simulink model "flex2"  (R2021b)
settings: Solver=ode1  StartTime=0.0  StopTime=4  FixedStep=0.001  RelTol=1e-3  EnableMultiTasking=on
values from neighbouring files (symbols this model uses):
  b1 = 0.0085    [part4_prelab.m]    (also in simulation_vs_exp.m; simulation_vs_exp_3_1.m; simulation_vs_exp_3_2.m; simulation_vs_exp_3_3.m)
  b2 = 8.4745E-4    (= 0.00084745)    [part4_prelab.m]    (also in simulation_vs_exp.m; simulation_vs_exp_3_1.m; simulation_vs_exp_3_2.m; simulation_vs_exp_3_3.m)
  c = 4.2    [part4_prelab.m]    (also in simulation_vs_exp.m = 0; simulation_vs_exp_3_1.m = 0; simulation_vs_exp_3_2.m = 0; simulation_vs_exp_3_3.m = 0)
  d1 = 0.5934    [simulation_vs_exp_3_1.m]    (also in simulation_vs_exp_3_2.m; simulation_vs_exp_3_3.m)
  d2 = 0.05934    [simulation_vs_exp_3_1.m]    (also in simulation_vs_exp_3_2.m; simulation_vs_exp_3_3.m)
  k = 0.0351    [part4_prelab.m]    (also in simulation_vs_exp.m; simulation_vs_exp_3_1.m; simulation_vs_exp_3_2.m; simulation_vs_exp_3_3.m)
  kp_notch = 1/amp    [simulation_vs_exp.m]    (also in simulation_vs_exp_3_1.m; simulation_vs_exp_3_2.m; simulation_vs_exp_3_3.m)
  m1 = 2.6634E-4    (= 0.00026634)    [part4_prelab.m]    (also in simulation_vs_exp.m; simulation_vs_exp_3_1.m; simulation_vs_exp_3_2.m; simulation_vs_exp_3_3.m)
  m2 = 1.4383E-4    (= 0.00014383)    [part4_prelab.m]    (also in simulation_vs_exp.m; simulation_vs_exp_3_1.m; simulation_vs_exp_3_2.m; simulation_vs_exp_3_3.m)
  wn = 17.33    [part4_prelab.m]    (also in simulation_vs_exp.m; simulation_vs_exp_3_1.m; simulation_vs_exp_3_2.m; simulation_vs_exp_3_3.m)
  zeta = 0.2669    [part4_prelab.m]    (also in simulation_vs_exp.m; simulation_vs_exp_3_1.m; simulation_vs_exp_3_2.m; simulation_vs_exp_3_3.m)
  zeta_den = 1    [part4_prelab.m]    (also in simulation_vs_exp.m; simulation_vs_exp_3_1.m; simulation_vs_exp_3_2.m; simulation_vs_exp_3_3.m)
undefined symbols (not defined in the file or in its folder): sgn, Ts
libraries: simulink x1
settings Model: SimulationMode=external  ExtModeTrigDuration=50000  Creator=mte360  LastModifiedBy=parth
settings SolverCC: AlgebraicLoopSolver=TrustRegion  PositivePriorityOrder=on
settings DataIOCC: LimitDataPoints=on  MaxDataPoints=100000  SaveFormat=Array  SignalLoggingSaveFormat=ModelDataLogs  ReturnWorkspaceOutputs=off
settings OptimizationCC: ExpressionDepthLimit=2147483647
settings DebuggingCC: UnderspecifiedInitializationDetection=Classic  MergeDetectMultiDrivingBlocksExec=none  SolverPrmCheckMsg=warning  FcnCallInpInsideContextMsg=warning  AllowSymbolicDim=off  StateNameClashWarn=warning  SFUnexpectedBacktrackingDiag=warning  SFNoUnconditionalDefaultTransitionDiag=warning  SFExecutionAtInitializationDiag=none  SFMachineParentedDataDiag=warning  ArithmeticOperatorsInVariantConditions=warning
settings ModelReferenceCC: PropagateSignalLabelsOutOfModel=off
settings SFSimCC: SimUseLocalCustomCode=off  CustomCodeUndefinedFunction=UseInterfaceOnly
settings RTWCC: Description=QUARC Win64 Target Using Toolchain  SystemTargetFile=quarc_win64.tlc  TemplateMakefile=quarc_default_tmf  RTWUseLocalCustomCode=off  Toolchain=QUARC win64 | nmake (64-bit Windows)  BuildConfiguration=Faster Runs
settings CodeAppCC: StateflowObjectComments=on
settings STFCustomTargetCC: ConcurrentExecutionCompliant=on  UseToolchainInfoCompliant=on  SystemTargetFile=quarc_win64.tlc
settings GRTTargetCC: TargetLangStandard=C89/C90 (ANSI)  ParMdlRefBuildCompliant=off  CompOptLevelCompliant=off  CombineOutputUpdateFcns=off  MatFileLogging=off  CPPClassGenCompliant=off  GRTInterface=on  ExtMode=on  ExtModeMexFile=quarc_comm
settings ConfigComp: CovMetricSettings=dw  CovSaveCumulativeToWorkspaceVar=on  CovSaveSingleToWorkspaceVar=on  CovExternalEMLEnable=off

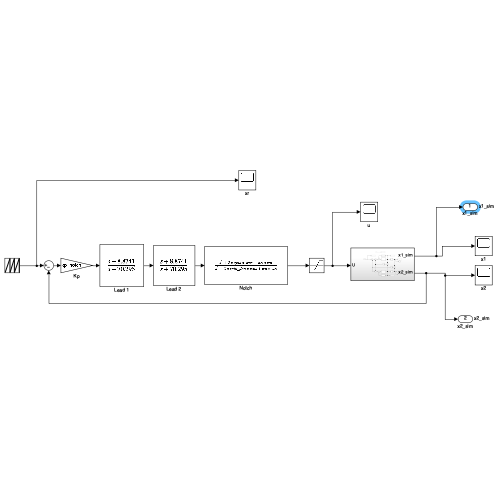
[thumbnail: Simulink's stored preview of the top-level diagram]
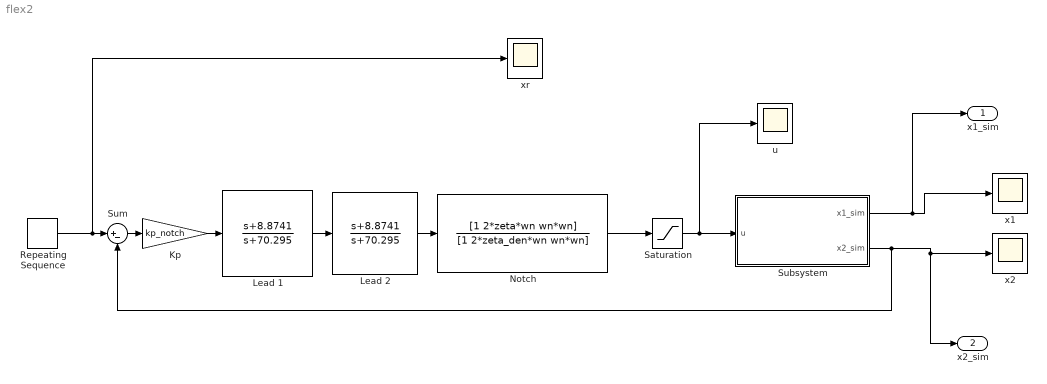
== system flex2 ==
  Kp : Gain  Gain=kp_notch
  Lead 1 : TransferFcn  Numerator=[1 8.8741]  Denominator=[1 70.295]
  Lead 2 : TransferFcn  Numerator=[1 8.8741]  Denominator=[1 70.295]
  Notch : TransferFcn  Numerator=[1 2*zeta*wn wn*wn]  Denominator=[1 2*zeta_den*wn wn*wn]
  Repeating Sequence : simulink/Sources/Repeating Sequence  rep_seq_t=t  rep_seq_y=s
  Saturation : Saturate  UpperLimit=8  LowerLimit=-8
  Subsystem : Subsystem
  Sum : Sum  Inputs=|+-
  u : Scope
  x1 : Scope
  x2 : Scope
  xr : Scope
  x1_sim : Outport  SignalName=x1_sim
  x2_sim : Outport  Port=2  SignalName=x2_sim
  wires:
  Repeating Sequence/1 -> xr/1, Sum/1
  Sum/1 -> Kp/1
  Kp/1 -> Lead 1/1
  Lead 1/1 -> Lead 2/1
  Lead 2/1 -> Notch/1
  Notch/1 -> Saturation/1
  Saturation/1 -> Subsystem/1(u), u/1
  Subsystem/1(x1_sim) -> x1/1, x1_sim/1
  Subsystem/2(x2_sim) -> x2_sim/1, x2/1, Sum/2

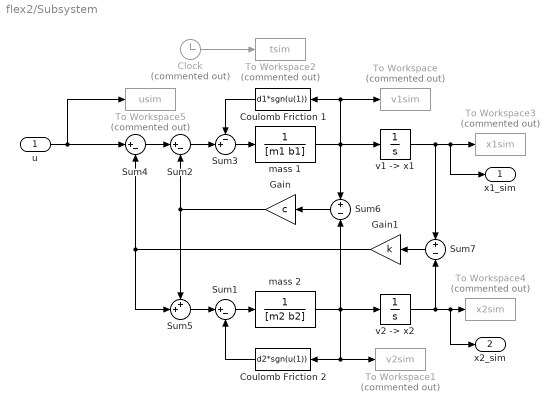
== system flex2/Subsystem ==
  u : Inport
  Clock : Clock  Commented=on
  Coulomb Friction 1 : Fcn  Expr=d1*sgn(u(1))
  Coulomb Friction 2 : Fcn  Expr=d2*sgn(u(1))
  Gain : Gain  Gain=c  SaturateOnIntegerOverflow=on  OutDataTypeStr=Inherit: Same as input  ParamDataTypeStr=Inherit: Same as input
  Gain1 : Gain  Gain=k  SaturateOnIntegerOverflow=on  OutDataTypeStr=Inherit: Same as input  ParamDataTypeStr=Inherit: Same as input
  Sum1 : Sum  Inputs=|+-  SaturateOnIntegerOverflow=on
  Sum2 : Sum  Inputs=|+-  SaturateOnIntegerOverflow=on
  Sum3 : Sum  Inputs=-+|  SaturateOnIntegerOverflow=on
  Sum4 : Sum  Inputs=|+-  SaturateOnIntegerOverflow=on
  Sum5 : Sum  Inputs=++|  SaturateOnIntegerOverflow=on
  Sum6 : Sum  Inputs=+|-  SaturateOnIntegerOverflow=on
  Sum7 : Sum  Inputs=+|-  SaturateOnIntegerOverflow=on
  To Workspace : ToWorkspace  Commented=on  VariableName=v1sim  SampleTime=Ts
  To Workspace1 : ToWorkspace  Commented=on  VariableName=v2sim  SampleTime=Ts
  To Workspace2 : ToWorkspace  Commented=on  VariableName=tsim  SampleTime=Ts
  To Workspace3 : ToWorkspace  Commented=on  VariableName=x1sim  SampleTime=Ts
  To Workspace4 : ToWorkspace  Commented=on  VariableName=x2sim  SampleTime=Ts
  To Workspace5 : ToWorkspace  Commented=on  VariableName=usim  SampleTime=Ts
  mass 1 : TransferFcn  Denominator=[m1 b1]
  mass 2 : TransferFcn  Denominator=[m2 b2]
  "v1 -> x1" : Integrator
  "v2 -> x2" : Integrator
  x1_sim : Outport
  x2_sim : Outport  Port=2
  wires:
  Sum5/1 -> Sum1/1
  Coulomb Friction 1/1 -> Sum3/1
  mass 1/1 -> "v1 -> x1"/1, Sum6/1, Coulomb Friction 1/1, To Workspace/1
  Gain/1 -> Sum2/2, Sum5/1
  Sum2/1 -> Sum3/2
  Sum3/1 -> mass 1/1
  Sum4/1 -> Sum2/1
  mass 2/1 -> "v2 -> x2"/1, Sum6/2, Coulomb Friction 2/1, To Workspace1/1
  Coulomb Friction 2/1 -> Sum1/2
  Sum6/1 -> Gain/1
  Gain1/1 -> Sum4/2, Sum5/2
  Sum1/1 -> mass 2/1
  "v1 -> x1"/1 -> Sum7/1, x1_sim/1, To Workspace3/1
  Sum7/1 -> Gain1/1
  Clock/1 -> To Workspace2/1
  "v2 -> x2"/1 -> Sum7/2, x2_sim/1, To Workspace4/1
  u/1 -> To Workspace5/1, Sum4/1
